simulink library "RWS"  (R2018a)
settings: Solver=ode45  StartTime=0.0  StopTime=10.0  RelTol=1e-3
undefined symbols (not defined in the file): ConfParam
libraries: simulink x3, SingleRWS x1
settings Model: Creator=y.akisheva  LastModifiedBy=Cédric
settings DataIOCC: LimitDataPoints=on  SaveFormat=Array
settings OptimizationCC: BlockReduction=off  BooleanDataType=off  LifeSpan=inf
settings DebuggingCC: SaveWithParameterizedLinksMsg=none  UnderspecifiedInitializationDetection=Classic  MergeDetectMultiDrivingBlocksExec=none  SignalResolutionControl=TryResolveAllWithWarning  SFUnexpectedBacktrackingDiag=warning  SFNoUnconditionalDefaultTransitionDiag=warning  SFExecutionAtInitializationDiag=none
settings HardwareCC: ProdBitPerPointer=32  ProdBitPerSizeT=32  ProdBitPerPtrDiffT=32  ProdLargestAtomicFloat=None  ProdIntDivRoundTo=Undefined  ProdEndianess=Unspecified  ProdWordSize=32  ProdHWDeviceType=32-bit Generic  TargetUnknown=on
settings ModelReferenceCC: PropagateSignalLabelsOutOfModel=off
settings CodeAppCC: StateflowObjectComments=on
settings GRTTargetCC: TargetLangStandard=C89/C90 (ANSI)  GeneratePreprocessorConditionals=Disable all
settings ConfigComp: CovMetricSettings=dw  CovHtmlReporting=on  CovSaveCumulativeToWorkspaceVar=on  CovSaveSingleToWorkspaceVar=on  CovExternalEMLEnable=off  CovSFcnEnable=off

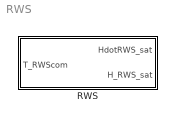
== system RWS ==
  RWS : Subsystem

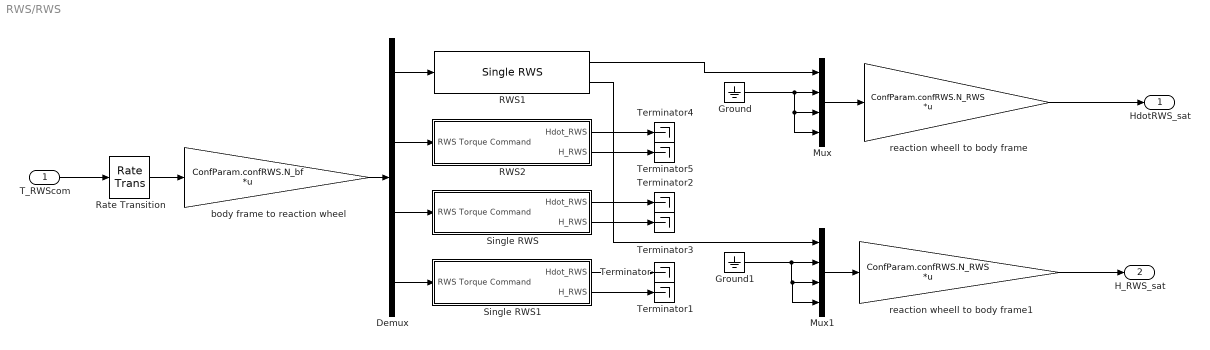
== system RWS/RWS ==
  T_RWScom : Inport
  Demux : Demux
  Ground : Ground
  Ground1 : Ground
  Mux : Mux
  Mux1 : Mux
  RWS1 : SingleRWS/Single RWS
  RWS2 : Subsystem
  Rate Transition : RateTransition  InitialCondition=[0;0;0]  OutPortSampleTime=ConfParam.confOrbit.dt
  Single RWS : Subsystem
  Single RWS1 : Subsystem
  Terminator{,1..5} (6 alike) : Terminator
  body frame to reaction wheel : Gain  Gain=ConfParam.confRWS.N_bf  Multiplication=Matrix(K*u)
  reaction wheell to body frame : Gain  Gain=ConfParam.confRWS.N_RWS  Multiplication=Matrix(K*u)
  reaction wheell to body frame1 : Gain  Gain=ConfParam.confRWS.N_RWS  Multiplication=Matrix(K*u)
  HdotRWS_sat : Outport
  H_RWS_sat : Outport  Port=2
  wires:
  Rate Transition/1 -> body frame to reaction wheel/1
  T_RWScom/1 -> Rate Transition/1
  body frame to reaction wheel/1 -> Demux/1
  Demux/1 -> RWS1/1
  Mux/1 -> reaction wheell to body frame/1
  RWS1/2 -> Mux1/1
  reaction wheell to body frame1/1 -> H_RWS_sat/1
  reaction wheell to body frame/1 -> HdotRWS_sat/1
  RWS1/1 -> Mux/1
  Demux/3 -> Single RWS/1(RWS Torque Command)
  Demux/4 -> Single RWS1/1(RWS Torque Command)
  Demux/2 -> RWS2/1(RWS Torque Command)
  Mux1/1 -> reaction wheell to body frame1/1
  Single RWS1/1(Hdot_RWS) -> Terminator/1
  Single RWS1/2(H_RWS) -> Terminator1/1
  Single RWS/1(Hdot_RWS) -> Terminator2/1
  Single RWS/2(H_RWS) -> Terminator3/1
  RWS2/1(Hdot_RWS) -> Terminator4/1
  RWS2/2(H_RWS) -> Terminator5/1
  Ground/1 -> Mux/4, Mux/3, Mux/2
  Ground1/1 -> Mux1/4, Mux1/3, Mux1/2

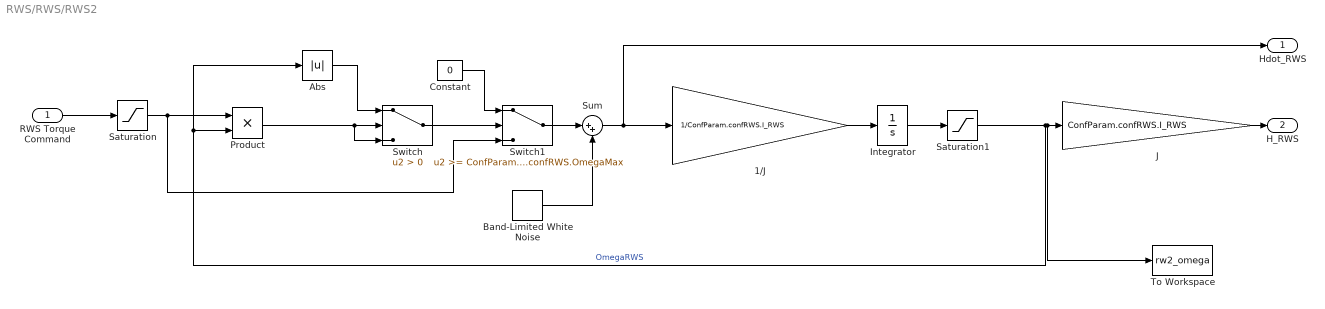
== system RWS/RWS/RWS2 ==
  RWS Torque Command : Inport
  1/J : Gain  Gain=1/ConfParam.confRWS.I_RWS
  Abs : Abs
  Band-Limited White Noise : simulink/Sources/Band-Limited White Noise  Cov=ConfParam.confRWS.NoisePower  Ts=ConfParam.confOrbit.dt  seed=[23341]
  Constant : Constant  Value=0
  Integrator : Integrator  InitialCondition=ConfParam.confRWS.IntitOmegaRWS(2)
  J : Gain  Gain=ConfParam.confRWS.I_RWS
  Product : Product
  Saturation : Saturate  UpperLimit=ConfParam.confRWS.Tmax  LowerLimit=-ConfParam.confRWS.Tmax
  Saturation1 : Saturate  UpperLimit=ConfParam.confRWS.OmegaMax  LowerLimit=-ConfParam.confRWS.OmegaMax
  Sum : Sum  Inputs=|++
  Switch : Switch  Criteria=u2 > Threshold
  Switch1 : Switch  Threshold=ConfParam.confRWS.OmegaMax
  To Workspace : ToWorkspace  VariableName=rw2_omega  SampleTime=-1
  Hdot_RWS : Outport
  H_RWS : Outport  Port=2
  wires:
  Band-Limited White Noise/1 -> Sum/2
  J/1 -> H_RWS/1
  Abs/1 -> Switch/1
  1/J/1 -> Integrator/1
  Sum/1 -> 1/J/1, Hdot_RWS/1
  Saturation1/1 -> J/1, To Workspace/1, Product/2, Abs/1  "OmegaRWS"
  Integrator/1 -> Saturation1/1
  Saturation/1 -> Switch1/3, Product/1
  Product/1 -> Switch/3, Switch/2
  RWS Torque Command/1 -> Saturation/1
  Constant/1 -> Switch1/1
  Switch/1 -> Switch1/2
  Switch1/1 -> Sum/1

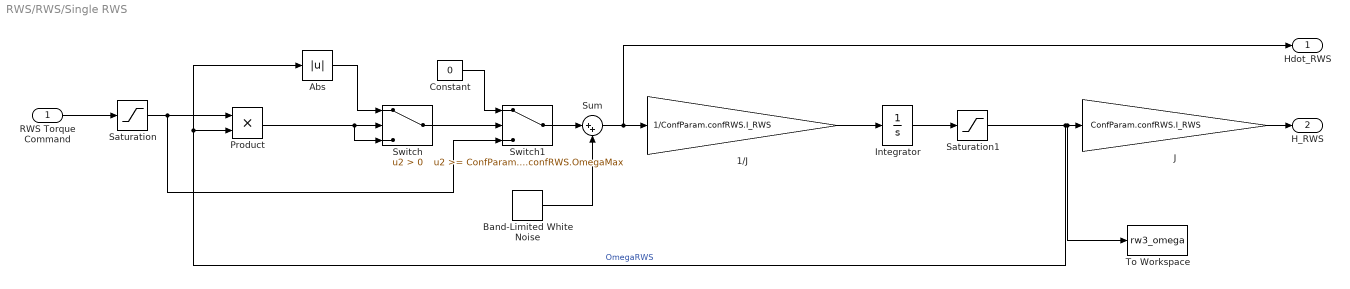
== system RWS/RWS/Single RWS ==
  RWS Torque Command : Inport
  1/J : Gain  Gain=1/ConfParam.confRWS.I_RWS
  Abs : Abs
  Band-Limited White Noise : simulink/Sources/Band-Limited White Noise  Cov=ConfParam.confRWS.NoisePower  Ts=ConfParam.confOrbit.dt  seed=[23341]
  Constant : Constant  Value=0
  Integrator : Integrator  InitialCondition=ConfParam.confRWS.IntitOmegaRWS(3)
  J : Gain  Gain=ConfParam.confRWS.I_RWS
  Product : Product
  Saturation : Saturate  UpperLimit=ConfParam.confRWS.Tmax  LowerLimit=-ConfParam.confRWS.Tmax
  Saturation1 : Saturate  UpperLimit=ConfParam.confRWS.OmegaMax  LowerLimit=-ConfParam.confRWS.OmegaMax
  Sum : Sum  Inputs=|++
  Switch : Switch  Criteria=u2 > Threshold
  Switch1 : Switch  Threshold=ConfParam.confRWS.OmegaMax
  To Workspace : ToWorkspace  VariableName=rw3_omega  SampleTime=-1
  Hdot_RWS : Outport
  H_RWS : Outport  Port=2
  wires:
  Band-Limited White Noise/1 -> Sum/2
  J/1 -> H_RWS/1
  Abs/1 -> Switch/1
  1/J/1 -> Integrator/1
  Sum/1 -> 1/J/1, Hdot_RWS/1
  Saturation1/1 -> Product/2, Abs/1, J/1, To Workspace/1  "OmegaRWS"
  Integrator/1 -> Saturation1/1
  Saturation/1 -> Switch1/3, Product/1
  Product/1 -> Switch/3, Switch/2
  RWS Torque Command/1 -> Saturation/1
  Constant/1 -> Switch1/1
  Switch/1 -> Switch1/2
  Switch1/1 -> Sum/1

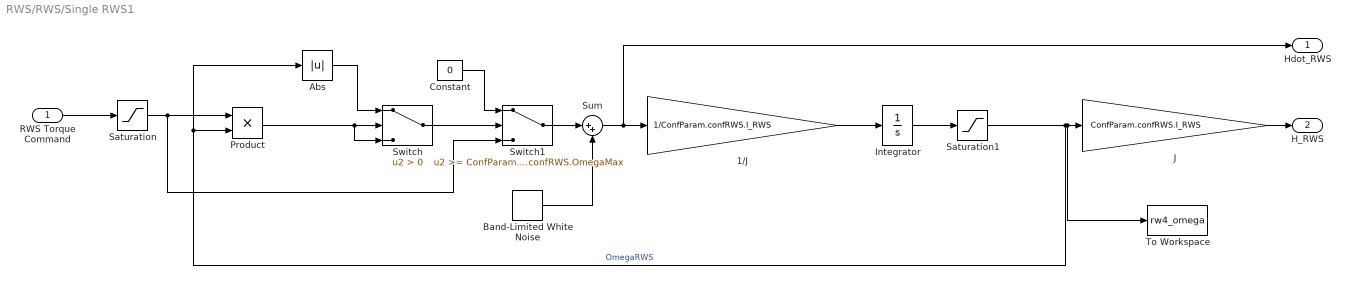
== system RWS/RWS/Single RWS1 ==
  RWS Torque Command : Inport
  1/J : Gain  Gain=1/ConfParam.confRWS.I_RWS
  Abs : Abs
  Band-Limited White Noise : simulink/Sources/Band-Limited White Noise  Cov=ConfParam.confRWS.NoisePower  Ts=ConfParam.confOrbit.dt  seed=[23341]
  Constant : Constant  Value=0
  Integrator : Integrator  InitialCondition=ConfParam.confRWS.IntitOmegaRWS(4)
  J : Gain  Gain=ConfParam.confRWS.I_RWS
  Product : Product
  Saturation : Saturate  UpperLimit=ConfParam.confRWS.Tmax  LowerLimit=-ConfParam.confRWS.Tmax
  Saturation1 : Saturate  UpperLimit=ConfParam.confRWS.OmegaMax  LowerLimit=-ConfParam.confRWS.OmegaMax
  Sum : Sum  Inputs=|++
  Switch : Switch  Criteria=u2 > Threshold
  Switch1 : Switch  Threshold=ConfParam.confRWS.OmegaMax
  To Workspace : ToWorkspace  VariableName=rw4_omega  SampleTime=-1
  Hdot_RWS : Outport
  H_RWS : Outport  Port=2
  wires:
  Band-Limited White Noise/1 -> Sum/2
  J/1 -> H_RWS/1
  Abs/1 -> Switch/1
  1/J/1 -> Integrator/1
  Sum/1 -> 1/J/1, Hdot_RWS/1
  Saturation1/1 -> Product/2, Abs/1, J/1, To Workspace/1  "OmegaRWS"
  Integrator/1 -> Saturation1/1
  Saturation/1 -> Switch1/3, Product/1
  Product/1 -> Switch/3, Switch/2
  RWS Torque Command/1 -> Saturation/1
  Constant/1 -> Switch1/1
  Switch/1 -> Switch1/2
  Switch1/1 -> Sum/1
